simulink model "MIMO3x3_model"  (R2018b)
settings: Solver=FixedStepAuto  StartTime=0.0  StopTime=Tmod  FixedStep=0.01  RelTol=1e-3
values from neighbouring files (symbols this model uses):
  denominator11 = FormDenominator(T1_11, T2_11, T3_11, flag11)    [Graph.m]    (also in KombRegNominalOU.m = FormDenominator(T1, T2, T3, flag); KombRobAdReg.m; KombRobReg.m; MIMONominalReg.m)
  denominator12 = FormDenominator(T1_12, T2_12, T3_12, flag12)    [Graph.m]    (also in KombRegNominalOU.m = FormDenominator(T1, T2, T3, flag); KombRobAdReg.m; KombRobReg.m; MIMONominalReg.m)
  denominator13 = FormDenominator(T1_13, T2_13, T3_13, flag13)    [Graph.m]    (also in KombRegNominalOU.m = FormDenominator(T1, T2, T3, flag); KombRobAdReg.m; KombRobReg.m; MIMONominalReg.m)
  denominator21 = FormDenominator(T1_21, T2_21, T3_21, flag21)    [Graph.m]    (also in KombRegNominalOU.m = FormDenominator(T1, T2, T3, flag); KombRobAdReg.m; KombRobReg.m; MIMONominalReg.m)
  denominator22 = FormDenominator(T1_22, T2_22, T3_22, flag22)    [Graph.m]    (also in KombRegNominalOU.m = FormDenominator(T1, T2, T3, flag); KombRobAdReg.m; KombRobReg.m; MIMONominalReg.m)
  denominator23 = FormDenominator(T1_23, T2_23, T3_23, flag23)    [Graph.m]    (also in KombRegNominalOU.m = FormDenominator(T1, T2, T3, flag); KombRobAdReg.m; KombRobReg.m; MIMONominalReg.m)
  denominator31 = FormDenominator(T1_31, T2_31, T3_31, flag31)    [Graph.m]    (also in KombRegNominalOU.m = FormDenominator(T1, T2, T3, flag); KombRobAdReg.m; KombRobReg.m; MIMONominalReg.m)
  denominator32 = FormDenominator(T1_32, T2_32, T3_32, flag32)    [Graph.m]    (also in KombRegNominalOU.m = FormDenominator(T1, T2, T3, flag); KombRobAdReg.m; KombRobReg.m; MIMONominalReg.m)
  denominator33 = FormDenominator(T1_33, T2_33, T3_33, flag33)    [Graph.m]    (also in KombRegNominalOU.m = FormDenominator(T1, T2, T3, flag); KombRobAdReg.m; KombRobReg.m; MIMONominalReg.m)
  ki11 = handles.savedValueWkiMS(1, 1)    [Graph.m]    (also in KombRegNominalOU.m = (ro_min *  (Wavt_Ki_Nom(1,1))) + ((1 - ro_min) * (Wvsp_Kp_No; KombRobAdReg.m = Wki_robast(1,1); KombRobReg.m = (ro_min_max *  (Wavt_Ki_Rob(1,1))) + ((1 - ro_min_max) * (Wv; MIMONominalReg.m = Wki_nominal(1,1))
  ki12 = handles.savedValueWkiMS(1, 2)    [Graph.m]    (also in KombRegNominalOU.m = (1 - ro_min) * (Wvsp_Ki_Nom(1,2)); KombRobAdReg.m = Wki_robast(1,2); KombRobReg.m = (1 - ro_min_max) * (Wvsp_Ki_Rob(1,2)); MIMONominalReg.m = Wki_nominal(1,2))
  ki13 = handles.savedValue7(1, 3)    [Graph.m]    (also in KombRegNominalOU.m = (ro_min *  (Wavt_Ki_Nom(1,3))) + ((1 - ro_min) * (Wvsp_Kp_No; KombRobAdReg.m = Wki_robast(1,3); KombRobReg.m = (1 - ro_min_max) * Wvsp_Ki_Rob(1, 3); MIMONominalReg.m = Wki_nominal(1,3))
  ki21 = handles.savedValueWkiMS(2, 1)    [Graph.m]    (also in KombRegNominalOU.m = (1 - ro_min) * (Wvsp_Ki_Nom(2,1)); KombRobAdReg.m = Wki_robast(2,1); KombRobReg.m = (1 - ro_min_max) * (Wvsp_Ki_Rob(2,1)); MIMONominalReg.m = Wki_nominal(2,1))
  ki22 = handles.savedValueWkiMS(2, 2)    [Graph.m]    (also in KombRegNominalOU.m = ro_min * (Wavt_Ki_Nom(2,2)) + ((1 - ro_min) * (Wvsp_Ki_Nom(2; KombRobAdReg.m = Wki_robast(2,2); KombRobReg.m = ro_min_max * (Wavt_Ki_Rob(2,2)) + ((1 - ro_min_max) * (Wvsp_; MIMONominalReg.m = Wki_nominal(2,2))
  ki23 = handles.savedValue7(2, 3)    [Graph.m]    (also in KombRegNominalOU.m = (ro_min *  (Wavt_Ki_Nom(2,3))) + ((1 - ro_min) * (Wvsp_Kp_No; KombRobAdReg.m = Wki_robast(2,3); KombRobReg.m = (1 - ro_min_max) * Wvsp_Ki_Rob(2,3); MIMONominalReg.m = Wki_nominal(2,3))
  ki31 = handles.savedValue7(3, 1)    [Graph.m]    (also in KombRegNominalOU.m = (ro_min *  (Wavt_Ki_Nom(3,1))) + ((1 - ro_min) * (Wvsp_Kp_No; KombRobAdReg.m = Wki_robast(3,1); KombRobReg.m = (1 - ro_min_max) * Wvsp_Ki_Rob(3,1); MIMONominalReg.m = Wki_nominal(3,1))
  ki32 = handles.savedValue7(3, 2)    [Graph.m]    (also in KombRegNominalOU.m = (ro_min *  (Wavt_Ki_Nom(3,2))) + ((1 - ro_min) * (Wvsp_Kp_No; KombRobAdReg.m = Wki_robast(3,2); KombRobReg.m = (1 - ro_min_max) * Wvsp_Ki_Rob(3,2); MIMONominalReg.m = Wki_nominal(3,2))
  ki33 = handles.savedValue7(3, 3)    [Graph.m]    (also in KombRegNominalOU.m = (ro_min *  (Wavt_Ki_Nom(3,3))) + ((1 - ro_min) * (Wvsp_Kp_No; KombRobAdReg.m = Wki_robast(3,3); KombRobReg.m = (ro_min_max * Wavt_Ki_Rob(3,3)) + ((1 - ro_min_max) * Wvsp_K; MIMONominalReg.m = Wki_nominal(3,3))
  kp11 = handles.savedValueWkpMS(1, 1)    [Graph.m]    (also in KombRegNominalOU.m = (ro_min * (Wavt_Kp_Nom(1,1))) + ((1 - ro_min) * (Wvsp_Kp_Nom; KombRobAdReg.m = Wkp_robast(1,1); KombRobReg.m = (ro_min_max * (Wavt_Kp_Rob(1,1))) + ((1 - ro_min_max) * (Wvs; MIMONominalReg.m = Wkp_nominal(1,1))
  kp12 = handles.savedValueWkpMS(1, 2)    [Graph.m]    (also in KombRegNominalOU.m = (1 - ro_min) * (Wvsp_Kp_Nom(1,2)); KombRobAdReg.m = Wkp_robast(1,2); KombRobReg.m = (1 - ro_min_max) * (Wvsp_Kp_Rob(1,2)); MIMONominalReg.m = Wkp_nominal(1,2))
  kp13 = handles.savedValue6(1, 3)    [Graph.m]    (also in KombRegNominalOU.m = (ro_min * (Wavt_Kp_Nom(1,3))) + ((1 - ro_min) * (Wvsp_Kp_Nom; KombRobAdReg.m = Wkp_robast(1,3); KombRobReg.m = (1 - ro_min_max) * Wvsp_Kp_Rob(1, 3); MIMONominalReg.m = Wkp_nominal(1,3))
  kp21 = handles.savedValueWkpMS(2, 1)    [Graph.m]    (also in KombRegNominalOU.m = (1 - ro_min) * (Wvsp_Kp_Nom(2,1)); KombRobAdReg.m = Wkp_robast(2,1); KombRobReg.m = (1 - ro_min_max) * (Wvsp_Kp_Rob(2,1)); MIMONominalReg.m = Wkp_nominal(2,1))
  kp22 = handles.savedValueWkpMS(2, 2)    [Graph.m]    (also in KombRegNominalOU.m = ro_min * (Wavt_Kp_Nom(2,2)) + ((1 - ro_min) * (Wvsp_Kp_Nom(2; KombRobAdReg.m = Wkp_robast(2,2); KombRobReg.m = ro_min_max * (Wavt_Kp_Rob(2,2)) + ((1 - ro_min_max) * (Wvsp_; MIMONominalReg.m = Wkp_nominal(2,2))
  kp23 = handles.savedValue6(2, 3)    [Graph.m]    (also in KombRegNominalOU.m = (ro_min * (Wavt_Kp_Nom(2,3))) + ((1 - ro_min) * (Wvsp_Kp_Nom; KombRobAdReg.m = Wkp_robast(2,3); KombRobReg.m = (1 - ro_min_max) * Wvsp_Kp_Rob(2,3); MIMONominalReg.m = Wkp_nominal(2,3))
  kp31 = handles.savedValue6(3, 1)    [Graph.m]    (also in KombRegNominalOU.m = (ro_min * (Wavt_Kp_Nom(3,1))) + ((1 - ro_min) * (Wvsp_Kp_Nom; KombRobAdReg.m = Wkp_robast(3,1); KombRobReg.m = (1 - ro_min_max) * Wvsp_Kp_Rob(3,1); MIMONominalReg.m = Wkp_nominal(3,1))
  kp32 = handles.savedValue6(3, 2)    [Graph.m]    (also in KombRegNominalOU.m = (ro_min * (Wavt_Kp_Nom(3,2))) + ((1 - ro_min) * (Wvsp_Kp_Nom; KombRobAdReg.m = Wkp_robast(3,2); KombRobReg.m = (1 - ro_min_max) * Wvsp_Kp_Rob(3,2); MIMONominalReg.m = Wkp_nominal(3,2))
  kp33 = handles.savedValue6(3, 3)    [Graph.m]    (also in KombRegNominalOU.m = (ro_min * (Wavt_Kp_Nom(3,3))) + ((1 - ro_min) * (Wvsp_Kp_Nom; KombRobAdReg.m = Wkp_robast(3,3); KombRobReg.m = (ro_min_max * Wavt_Kp_Rob(3,3)) + ((1 - ro_min_max) * Wvsp_K; MIMONominalReg.m = Wkp_nominal(3,3))
  numerator11 = FormNumerator(k11, k11_2)    [Graph.m]    (also in KombRegNominalOU.m = FormNumerator(k, k2); KombRobAdReg.m; KombRobReg.m; MIMONominalReg.m)
  numerator12 = FormNumerator(k12, k12_2)    [Graph.m]    (also in KombRegNominalOU.m = FormNumerator(k, k2); KombRobAdReg.m; KombRobReg.m; MIMONominalReg.m)
  numerator13 = FormNumerator(k13, k13_2)    [Graph.m]    (also in KombRegNominalOU.m = FormNumerator(k, k2); KombRobAdReg.m; KombRobReg.m; MIMONominalReg.m)
  numerator21 = FormNumerator(k21, k21_2)    [Graph.m]    (also in KombRegNominalOU.m = FormNumerator(k, k2); KombRobAdReg.m; KombRobReg.m; MIMONominalReg.m)
  numerator22 = FormNumerator(k22, k22_2)    [Graph.m]    (also in KombRegNominalOU.m = FormNumerator(k, k2); KombRobAdReg.m; KombRobReg.m; MIMONominalReg.m)
  numerator23 = FormNumerator(k23, k23_2)    [Graph.m]    (also in KombRegNominalOU.m = FormNumerator(k, k2); KombRobAdReg.m; KombRobReg.m; MIMONominalReg.m)
  numerator31 = FormNumerator(k31, k31_2)    [Graph.m]    (also in KombRegNominalOU.m = FormNumerator(k, k2); KombRobAdReg.m; KombRobReg.m; MIMONominalReg.m)
  numerator32 = FormNumerator(k32, k32_2)    [Graph.m]    (also in KombRegNominalOU.m = FormNumerator(k, k2); KombRobAdReg.m; KombRobReg.m; MIMONominalReg.m)
  numerator33 = FormNumerator(k33, k33_2)    [Graph.m]    (also in KombRegNominalOU.m = FormNumerator(k, k2); KombRobAdReg.m; KombRobReg.m; MIMONominalReg.m)
  tau11 = tau11_grid(idx)    [KombRobAdReg.m]    (also in KombRobReg.m; MIMONominalReg.m)
  tau12 = tau12_grid(idx)    [KombRobAdReg.m]    (also in KombRobReg.m; MIMONominalReg.m)
  tau13 = tau13_grid(idx)    [KombRobAdReg.m]    (also in KombRobReg.m; MIMONominalReg.m)
  tau21 = tau21_grid(idx)    [KombRobAdReg.m]    (also in KombRobReg.m; MIMONominalReg.m)
  tau22 = tau22_grid(idx)    [KombRobAdReg.m]    (also in KombRobReg.m; MIMONominalReg.m)
  tau23 = tau23_grid(idx)    [KombRobAdReg.m]    (also in KombRobReg.m; MIMONominalReg.m)
  tau31 = tau31_grid(idx)    [KombRobAdReg.m]    (also in KombRobReg.m; MIMONominalReg.m)
  tau32 = tau32_grid(idx)    [KombRobAdReg.m]    (also in KombRobReg.m; MIMONominalReg.m)
  tau33 = tau33_grid(idx)    [KombRobAdReg.m]    (also in KombRobReg.m; MIMONominalReg.m)
  Tmod = 500    [Approximation.m]    (also in ApproximationUncertainty.m; Main.m = 100; MainMenu.m = numericValueTmod)
undefined symbols (not defined in the file or in its folder): disturbance1, disturbance2, disturbance3
settings Model: Creator=stepa  LastModifiedBy=stepa

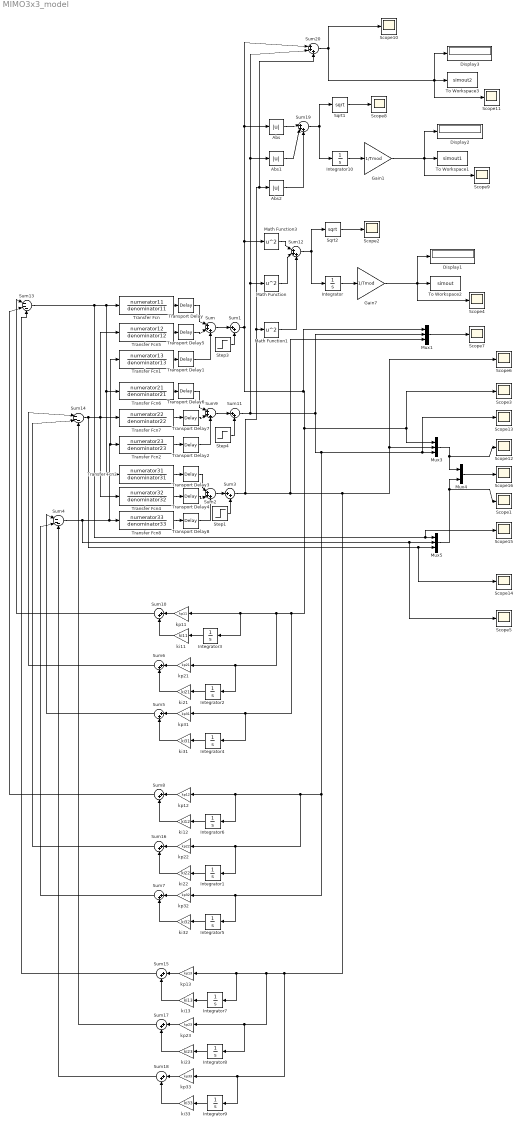
== system MIMO3x3_model ==
  Abs : Abs
  Abs1 : Abs
  Abs2 : Abs
  Display1 : Display
  Display2 : Display
  Display3 : Display
  Gain1 : Gain  Gain=1/Tmod
  Gain7 : Gain  Gain=1/Tmod
  Integrator{,1..10} (11 alike) : Integrator
  Math Function : Math  Operator=square  SaturateOnIntegerOverflow=on
  Math Function1 : Math  Operator=square  SaturateOnIntegerOverflow=on
  Math Function3 : Math  Operator=square  SaturateOnIntegerOverflow=on
  Mux1 : Mux  Inputs=3
  Mux3 : Mux  Inputs=3
  Mux4 : Mux  Inputs=2
  Mux5 : Mux  Inputs=3
  Scope{1..16} (16 alike) : Scope
  Sqrt1 : Sqrt  SaturateOnIntegerOverflow=on
  Sqrt2 : Sqrt  SaturateOnIntegerOverflow=on
  Step1 : Step  After=disturbance3  SampleTime=0
  Step3 : Step  After=disturbance1  SampleTime=0
  Step4 : Step  After=disturbance2  SampleTime=0
  Sum{,2,9,12,19..20} (6 alike) : Sum  Inputs=|+++
  Sum{1,3,5..8,10..11,15..18} (12 alike) : Sum  Inputs=|++
  Sum13 : Sum  Inputs=|---
  Sum14 : Sum  Inputs=|---
  Sum4 : Sum  Inputs=|---
  To Workspace1 : ToWorkspace  VariableName=simout1  SampleTime=-1
      settings: MaxDataPoints=1
  To Workspace2 : ToWorkspace  VariableName=simout  SampleTime=-1
      settings: MaxDataPoints=1
  To Workspace3 : ToWorkspace  VariableName=simout2  SampleTime=-1
      settings: MaxDataPoints=50000
  Transfer Fcn : TransferFcn  Numerator=numerator11  Denominator=denominator11
  Transfer Fcn1 : TransferFcn  Numerator=numerator13  Denominator=denominator13
  Transfer Fcn2 : TransferFcn  Numerator=numerator23  Denominator=denominator23
  Transfer Fcn3 : TransferFcn  Numerator=numerator31  Denominator=denominator31
  Transfer Fcn4 : TransferFcn  Numerator=numerator32  Denominator=denominator32
  Transfer Fcn5 : TransferFcn  Numerator=numerator12  Denominator=denominator12
  Transfer Fcn6 : TransferFcn  Numerator=numerator21  Denominator=denominator21
  Transfer Fcn7 : TransferFcn  Numerator=numerator22  Denominator=denominator22
  Transfer Fcn8 : TransferFcn  Numerator=numerator33  Denominator=denominator33
  Transport Delay : TransportDelay  DelayTime=tau11
  Transport Delay1 : TransportDelay  DelayTime=tau13
  Transport Delay2 : TransportDelay  DelayTime=tau23
  Transport Delay3 : TransportDelay  DelayTime=tau31
  Transport Delay4 : TransportDelay  DelayTime=tau32
  Transport Delay5 : TransportDelay  DelayTime=tau12
  Transport Delay6 : TransportDelay  DelayTime=tau21
  Transport Delay7 : TransportDelay  DelayTime=tau22
  Transport Delay8 : TransportDelay  DelayTime=tau33
  ki11 : Gain  Gain=ki11
  ki12 : Gain  Gain=ki12
  ki13 : Gain  Gain=ki13
  ki21 : Gain  Gain=ki21
  ki22 : Gain  Gain=ki22
  ki23 : Gain  Gain=ki23
  ki31 : Gain  Gain=ki31
  ki32 : Gain  Gain=ki32
  ki33 : Gain  Gain=ki33
  kp11 : Gain  Gain=kp11
  "kp12 " : Gain  Gain=kp12
  kp13 : Gain  Gain=kp13
  kp21 : Gain  Gain=kp21
  kp22 : Gain  Gain=kp22
  kp23 : Gain  Gain=kp23
  kp31 : Gain  Gain=kp31
  kp32 : Gain  Gain=kp32
  kp33 : Gain  Gain=kp33
  wires:
  Integrator8/1 -> ki23/1
  Sum10/1 -> Sum13/1
  Mux1/1 -> Scope7/1
  Transfer Fcn7/1 -> Transport Delay7/1
  ki33/1 -> Sum18/2
  Step4/1 -> Sum11/2
  Transport Delay3/1 -> Sum2/1
  Sum5/1 -> Sum4/1
  ki32/1 -> Sum7/2
  Sum12/1 -> Integrator/1, Sqrt2/1
  Sum15/1 -> Sum13/3
  Sum7/1 -> Sum4/2
  ki13/1 -> Sum15/2
  Transfer Fcn4/1 -> Transport Delay4/1
  Sum18/1 -> Sum4/3
  ki31/1 -> Sum5/2
  Transfer Fcn2/1 -> Transport Delay2/1
  Integrator/1 -> Gain7/1
  Sum17/1 -> Sum14/3
  kp22/1 -> Sum16/1
  Sum14/1 -> Transfer Fcn4/1, Transfer Fcn7/1, Transfer Fcn5/1, Mux5/3, Scope14/1
  Sum3/1 -> Sum20/3, Abs2/1, Math Function1/1, Mux1/3, Integrator9/1, kp33/1, kp23/1, Integrator8/1, Integrator7/1, kp13/1, Scope6/1, Mux3/2
  kp33/1 -> Sum18/1
  kp31/1 -> Sum5/1
  Integrator9/1 -> ki33/1
  Sum1/1 -> Mux1/1, Integrator4/1, kp31/1, Integrator3/1, kp11/1, Integrator2/1, kp21/1, Scope3/1, Mux3/1, Sum20/1, Abs/1, Math Function3/1
  Math Function/1 -> Sum12/2
  Transfer Fcn3/1 -> Transport Delay3/1
  Integrator4/1 -> ki31/1
  ki23/1 -> Sum17/2
  kp32/1 -> Sum7/1
  Step3/1 -> Sum1/2
  kp23/1 -> Sum17/1
  kp13/1 -> Sum15/1
  Sum11/1 -> Sum20/2, Abs1/1, Math Function/1, Mux1/2, Integrator5/1, kp32/1, "kp12 "/1, Integrator6/1, kp22/1, Integrator1/1, Scope13/1, Mux3/3
  Integrator6/1 -> ki12/1
  Transport Delay8/1 -> Sum2/3
  Math Function1/1 -> Sum12/3
  Sum13/1 -> Transfer Fcn/1, Transfer Fcn3/1, Transfer Fcn6/1, Scope15/1, Mux5/1
  kp21/1 -> Sum6/1
  ki21/1 -> Sum6/2
  Sum2/1 -> Sum3/1
  Integrator2/1 -> ki21/1
  Sum4/1 -> Scope5/1, Mux5/2, Transfer Fcn8/1, Transfer Fcn2/1, Transfer Fcn1/1
  Transfer Fcn/1 -> Transport Delay/1
  Step1/1 -> Sum3/2
  Transfer Fcn5/1 -> Transport Delay5/1
  Integrator7/1 -> ki13/1
  Integrator1/1 -> ki22/1
  Transport Delay4/1 -> Sum2/2
  Mux4/1 -> Scope16/1
  Sum/1 -> Sum1/1
  Integrator3/1 -> ki11/1
  Transport Delay6/1 -> Sum9/1
  Math Function3/1 -> Sum12/1
  Sum9/1 -> Sum11/1
  Transfer Fcn1/1 -> Transport Delay1/1
  Integrator5/1 -> ki32/1
  Transport Delay/1 -> Sum/1
  Mux3/1 -> Mux4/1, Scope12/1
  ki11/1 -> Sum10/2
  Mux5/1 -> Mux4/2, Scope1/1
  Sum8/1 -> Sum13/2
  Gain7/1 -> Scope4/1, Display1/1, To Workspace2/1
  Transport Delay5/1 -> Sum/2
  Transfer Fcn8/1 -> Transport Delay8/1
  Transport Delay7/1 -> Sum9/2
  "kp12 "/1 -> Sum8/1
  Sum16/1 -> Sum14/2
  Transport Delay2/1 -> Sum9/3
  Sum6/1 -> Sum14/1
  Sqrt2/1 -> Scope2/1
  Transfer Fcn6/1 -> Transport Delay6/1
  ki22/1 -> Sum16/2
  ki12/1 -> Sum8/2
  Transport Delay1/1 -> Sum/3
  kp11/1 -> Sum10/1
  Sqrt1/1 -> Scope8/1
  Abs1/1 -> Sum19/2
  Integrator10/1 -> Gain1/1
  Abs/1 -> Sum19/1
  Gain1/1 -> Scope9/1, To Workspace1/1, Display2/1
  Sum19/1 -> Integrator10/1, Sqrt1/1
  Abs2/1 -> Sum19/3
  Sum20/1 -> Scope11/1, To Workspace3/1, Display3/1, Scope10/1
